simulink model "lab0701"  (R2016a)
settings: Solver=VariableStepAuto  StartTime=0.0  StopTime=10.0  RelTol=1e-3
undefined symbols (not defined in the file): DiscIntNeverNeededParam
libraries: dspsrcs4 x1
settings Model: PauseTimes=0.2  Creator=Student  LastModifiedBy=Student

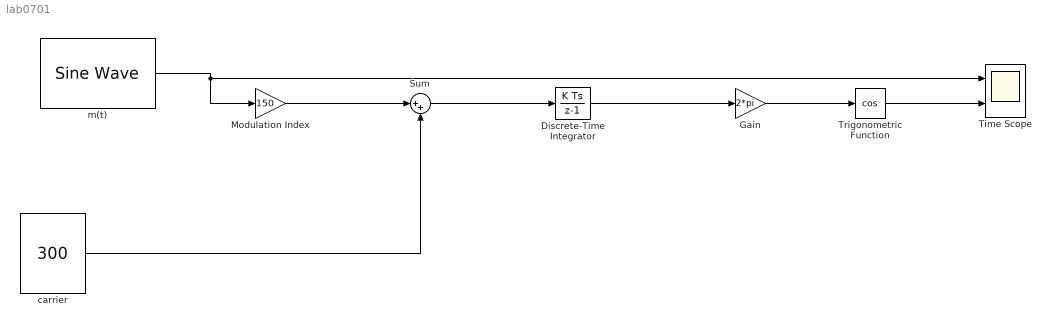
== system lab0701 ==
  Discrete-Time Integrator : DiscreteIntegrator  gainval=1  InitialConditionSetting=State (most efficient)  ICPrevOutput=DiscIntNeverNeededParam  ICPrevScaledInput=DiscIntNeverNeededParam
  Gain : Gain  Gain=2*pi
  Modulation Index : Gain  Gain=150
  Sum : Sum  Inputs=|++
  Time Scope : Scope  NumInputPorts=2
  Trigonometric Function : Trigonometry  Operator=cos
  "carrier " : Constant  Value=300
  "m(t) " : dspsrcs4/Sine Wave  Amplitude=1  Frequency=10  Phase=90  SampleMode=Discrete  OutComplex=Real  CompMethod=Trigonometric fcn  TableSize=Speed  SampleTime=1/98000  SamplesPerFrame=1  ResetState=Restart at time zero  OutputFrames=off  dataType=double  wordLen=16  udDataType=sfix(16)  fracBitsMode=Best precision  numFracBits=15  OutDataTypeStr=double  LastOutDataTypeStr=double
  wires:
  "m(t) "/1 -> Time Scope/1, Modulation Index/1
  Modulation Index/1 -> Sum/1
  Sum/1 -> Discrete-Time Integrator/1
  Discrete-Time Integrator/1 -> Gain/1
  Gain/1 -> Trigonometric Function/1
  Trigonometric Function/1 -> Time Scope/2
  "carrier "/1 -> Sum/2
